simulink model "openloop_model_control_synthesis_paper_SAuncertain"  (R2024a)
settings: Solver=VariableStepAuto  StartTime=0.0  StopTime=10.0  RelTol=1e-3
values from neighbouring files (symbols this model uses):
  a_ASD_GYRO = 9.1987e-04    (= 0.00091987)    [data.m]
  a_ASD_SST = 1.5343e-05    [data.m]
  APE = [50 50 50]'*9*0.001*pi/180    [data.m]
  Plant = ulinearize('SDT_USS_paper_SAuncertain')    [main.m]
libraries: cstblocks x6, RCTblocks x1
settings Model: Creator=T.FORMOSA  LastModifiedBy=r.de-oliveira
settings SolverCC: AlgebraicLoopSolver=TrustRegion
settings DebuggingCC: AlgebraicLoopMsg=none  UnconnectedInputMsg=warning  UnconnectedOutputMsg=warning  UnconnectedLineMsg=warning  ArithmeticOperatorsInVariantConditions=warning
settings ModelReferenceCC: EnableRefExpFcnMdlSchedulingChecks=on
settings SFSimCC: CustomCodeUndefinedFunction=UseInterfaceOnly
settings RTWCC: GPUComputeCapability=3.5  DLArmComputeVersion=19.05

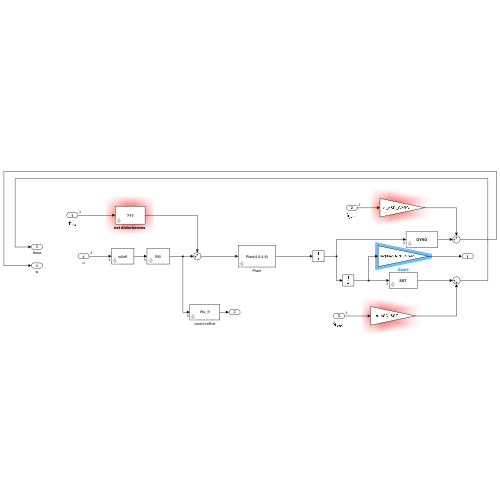
[thumbnail: Simulink's stored preview of the top-level diagram]
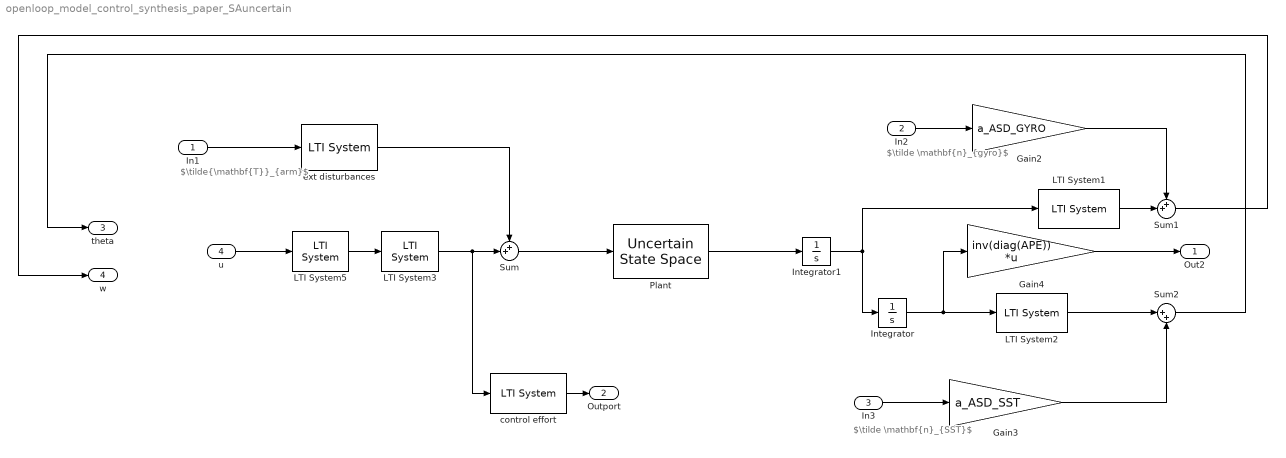
== system openloop_model_control_synthesis_paper_SAuncertain ==
  note: $\tilde \mathbf{n}_{SST}$
  note: $\tilde \mathbf{n}_{gyro}$
  note: $\tilde{\mathbf{T}}_{arm}$
  In1 : Inport  PortDimensions=3
  In2 : Inport  Port=2  PortDimensions=3
  In3 : Inport  Port=3  PortDimensions=3
  u : Inport  Port=4  PortDimensions=3
  Gain2 : Gain  Gain=a_ASD_GYRO
  Gain3 : Gain  Gain=a_ASD_SST
  Gain4 : Gain  Gain=inv(diag(APE))  Multiplication=Matrix(K*u) (u vector)
  Integrator : Integrator
  Integrator1 : Integrator
  LTI System1 : cstblocks/LTI System  sys=GYRO  IC=[]  PadeOrder=0
  LTI System2 : cstblocks/LTI System  sys=SST  IC=[]  PadeOrder=0
  LTI System3 : cstblocks/LTI System  sys=RW  IC=[]  PadeOrder=0
  LTI System5 : cstblocks/LTI System  sys=rolloff  IC=[]  PadeOrder=0
  Plant : RCTblocks/Uncertain State Space  Tag=USS  SCDEnableBlockLinearizationSpecification=on  USystem=Plant(4:6,4:6)  UValue=[]  X0=[]  uX0=[]
  Sum : Sum  Inputs=++|
  Sum1 : Sum  Inputs=++|
  Sum2 : Sum  Inputs=|++
  control effort : cstblocks/LTI System  sys=Wu_tf  IC=[]  PadeOrder=0
  "ext disturbances " : cstblocks/LTI System  sys=Htotcont  IC=[]  PadeOrder=0
  Out2 : Outport  VectorParamsAs1DForOutWhenUnconnected=off
  Outport : Outport  Port=2
  theta : Outport  Port=3
  w : Outport  Port=4
  wires:
  Integrator1/1 -> LTI System1/1, Integrator/1
  LTI System1/1 -> Sum1/2
  In2/1 -> Gain2/1
  Sum2/1 -> theta/1
  In3/1 -> Gain3/1
  LTI System2/1 -> Sum2/1
  Integrator/1 -> Gain4/1, LTI System2/1
  Sum1/1 -> w/1
  Sum/1 -> Plant/1
  "ext disturbances "/1 -> Sum/1
  Gain2/1 -> Sum1/1
  Gain3/1 -> Sum2/2
  In1/1 -> "ext disturbances "/1
  Plant/1 -> Integrator1/1
  Gain4/1 -> Out2/1
  u/1 -> LTI System5/1
  control effort/1 -> Outport/1
  LTI System5/1 -> LTI System3/1
  LTI System3/1 -> control effort/1, Sum/2
